simulink model "Rcontrol_veryold"  (Simulink 7.5)
settings: Solver=ode3  StartTime=0.0  StopTime=inf  FixedStep=SampleTime  RelTol=1e-3
undefined symbols (not defined in the file or in its folder): none, Rec, SampleTime, SDTV, videoinput
libraries: simulink x4, vipsnks x3, vipconversions x2, vipstatistics x1, viptextngfix x1, imaqlib x1, simulink_need_slupdate x1
settings Model: Creator=Duarte  LastModifiedBy=PC1
settings CodeAppCC: CustomSymbolStrType=$N$R$M_T
settings GRTTargetCC: TargetFunctionLibrary=NOT IN USE

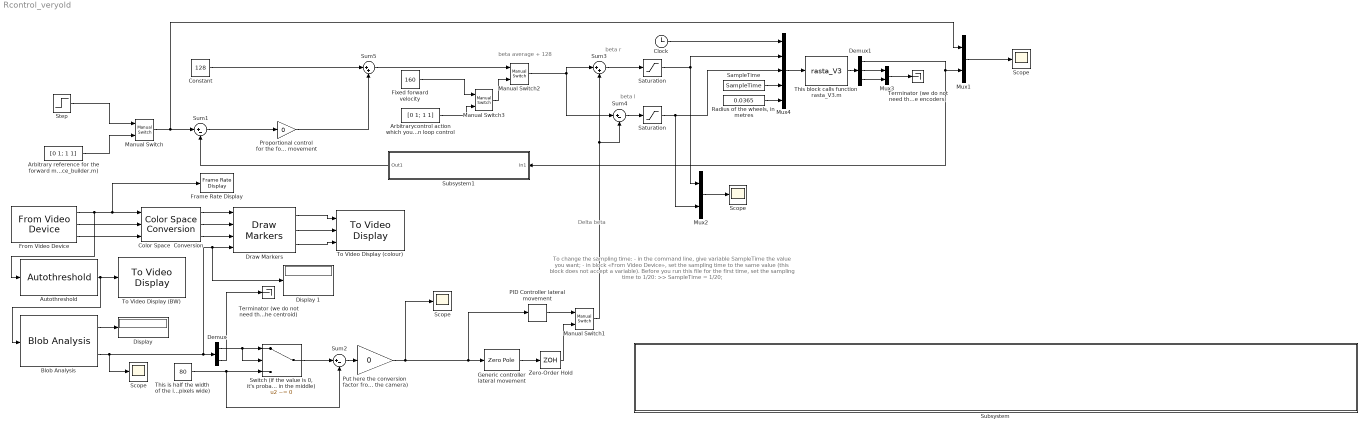
== system Rcontrol_veryold ==
  note: beta l
  note: beta r
  note: beta average + 128
  note: Delta beta
  note: To change the sampling time:
      | - in the command line, give variable SampleTime the value you want;
      | - in block «From Video Device», set the sampling time to the same value (this block does not accept a variable).
      | Before you run this file for the first time, set the sampling time to 1/20:
      |      >> SampleTime = 1/20;
  "Arbitrary reference for the forward movement, which you may change (use here the variable created by reference_builder.m)" : FromWorkspace  VariableName=[0 1; 1 1]  SampleTime=SampleTime
  Arbitrarycontrol action which you may use for open loop control : FromWorkspace  VariableName=[0 1; 1 1]  SampleTime=SampleTime
  Autothreshold : vipconversions/Autothreshold  DialogController=vipDDGCreate  DialogControllerArgs=DataTag0  operator=<=  threshOut=off  effMetricOut=off  userDefinedRange=off  umin=0  umax=255  outOfRngOpt=Warn and saturate  scaleThreshold=off  scaleFactor=1  P1Mode=Specify word length  P1WordLength=32  P1FracLength=30  P2Mode=Specify word length  P2WordLength=32  P2FracLength=22  P3Mode=Specify word length  P3WordLength=32  P3FracLength=14  P4Mode=Binary point scaling  P4WordLength=32  P4FracLength=15  Q1Mode=Specify word length  Q1WordLength=32  Q1FracLength=16  EMMode=Specify word length  EMWordLength=16  EMFracLength=14  roundingMode=Floor  overflowMode=off
  Blob Analysis : vipstatistics/Blob Analysis  Tag=vipblks_row_conv  DialogController=vipDDGCreate  DialogControllerArgs=DataTag1  area=on  centroid=on  bBox=off  majorAxis=off  minorAxis=off  angle=off  eccentricity=off  equivDiameterSq=off  extent=off  perimeter=off  maxBlobs=1  warnIfNumBlobsExceeded=off  isCount=off  useMinArea=off  minArea=0  useMaxArea=off  maxArea=intmax('uint32')  excludeBorderBlob=off  outDT=double  isOutVarDim=off  isFill=on  fillValues=-1  conn=8  isLabel=off  outputMode=Binary point scaling  outputWordLength=32  outputFracLength=16  firstCoeffMode=Binary point scaling  firstCoeffWordLength=16  firstCoeffFracLength=14  secondCoeffMode=Binary point scaling  secondCoeffWordLength=32  secondCoeffFracLength=16  accumMode=Binary point scaling  accumWordLength=32  accumFracLength=0  prodOutputMode=Binary point scaling  prodOutputWordLength=32  prodOutputFracLength=16  roundingMode=Floor  overflowMode=off
  Clock : Clock
      settings: Decimation=10
  Color Space  Conversion : vipconversions/Color Space  Conversion  conversion=Obsolete  conversionActive=Y'CbCr to R'G'B'  wp_str=D65  rec=Rec. 601 (SDTV)  sys=1125/60/2:1  imagePorts=Separate color signals
  Constant : Constant  Value=128
  Demux : Demux  Outputs=2
  Demux1 : Demux  Outputs=3
  "Display " : Display
  Display 1 : Display
  Draw Markers : viptextngfix/Draw Markers  DialogController=vipDDGCreate  DialogControllerArgs=DataTag2  shape=Circle  size=5  fill=off  fillClrSource=Specify via dialog  display=User-specified value  intensity=200  color=[200 0 0]  opacity=0.6  viewport=Entire image  antialiasing=off  inType=Obsolete  imagePorts=Separate color signals  prodOutputMode=Binary point scaling  prodOutputWordLength=32  prodOutputFracLength=14  memoryMode=Specify word length  memoryWordLength=16  memoryFracLength=15  roundingMode=Floor  overflowMode=off
  Fixed forward velocity : Constant  Value=160
  Frame Rate Display : vipsnks/Frame Rate Display  DialogController=vipDDGCreate  DialogControllerArgs=DataTag3  UpdateRate=10
  From Video Device : imaqlib/From Video Device  DialogController=imaqcreatedialog  DialogControllerArgs=DataTag5  DeviceMenu=winvideo 2 (USB2.0 PC CAMERA)  Device=winvideo 2 (USB2.0 PC CAMERA)  ObjConstructor=videoinput('winvideo', 2)  VideoFormatMenu=YUY2_160x120  VideoFormat=YUY2_160x120  VideoSource=input1  ROIPosition=[0 0 120 160]  EnableHWTrigger=off  TriggerConfiguration=none/none  SampleTime=1/8  OutputPortsMode=Separate color signals  DataType=single  CanDoHWTrigger=no  ReturnedColorSpace=YCbCr  BlockHandle=17.001  ROIWidth=160  ROIHeight=120
  Generic controller lateral movement : ZeroPole  Zeros=[-1]  Poles=[-2]  Gain=1/3
  Manual Switch : simulink/Signal Routing/Manual Switch  SystemSampleTime=-1  sw=0  action=0  varsize=off
  Manual Switch1 : simulink/Signal Routing/Manual Switch  SystemSampleTime=-1  sw=1  action=0  varsize=off
  Manual Switch2 : simulink/Signal Routing/Manual Switch  SystemSampleTime=-1  sw=1  action=0  varsize=off
  Manual Switch3 : simulink/Signal Routing/Manual Switch  SystemSampleTime=-1  sw=1  action=0  varsize=off
  Mux1 : Mux  Inputs=2
  Mux2 : Mux  Inputs=2
  Mux3 : Mux  Inputs=2
  Mux4 : Mux  Inputs=5
  PID Controller lateral movement : simulink_need_slupdate/PID Controller  SystemSampleTime=-1  P=0  I=0  D=0
  Proportional control for the forward movement : Gain  Gain=0
  Put here the conversion factor from pixels to rad (this is the gain of the camera) : Gain  Gain=0
  "Radius of the wheels, in metres" : Constant  Value=0.0365
  SampleTime : Constant  Value=SampleTime
  Saturation : Saturate  UpperLimit=255  LowerLimit=0
  "Saturation " : Saturate  UpperLimit=255  LowerLimit=0
  Scope : Scope
      settings: YMin=0.985  YMax=1  SaveName=DataFwd
  "Scope  " : Scope
      settings: YMin=0  YMax=85  SaveName=DataCentr
  "Scope   " : Scope
      settings: SaveName=DataCtrl
  "Scope     " : Scope
      settings: SaveName=DataRotation
  Step : Step  Time=0  SampleTime=SampleTime
  Subsystem : Subsystem
      settings: OpenFcn=|
      | % find what ports have been open
      | whatsopen = instrfind;
      | for k = 1 : length(whatsopen)
      |     if strcmp( whatsopen(k).Status , 'open' )
      |         % if there's an open port...
      |         fclose(whatsopen(k));
      |         % ...close it
      |     end
      | end
      | % now we know everything's closed
      mask Display: disp('Double-click this block to close all the open ports')
  Subsystem1 : Subsystem
  Sum1 : Sum  Inputs=|+-
  Sum2 : Sum  Inputs=|+-
  Sum3 : Sum  Inputs=|++
  Sum4 : Sum  Inputs=|+-
  Sum5 : Sum  Inputs=|++
  "Switch (if the value is 0, it's probably a mistake, so assume it's in the middle)" : Switch  Criteria=u2 ~= 0
  Terminator (we do not need the values from the encoders) : Terminator
  Terminator (we do not need the y coordinate of the centroid) : Terminator
  This block calls function rasta_V3.m : MATLABFcn  MATLABFcn=rasta_V3  Output1D=off  SampleTime=SampleTime
  This is half the width of the image (change this if your image is not 160 pixels wide) : Constant  Value=80
  To Video Display (BW) : vipsnks/To Video Display  DialogControllerArgs=DataTag6  inputType=Obsolete  imagePorts=One multidimensional signal  OutputDevice=On-screen video monitor  fullScreen=off  videoWindowX=44  videoWindowY=27  saveWindowSize=off  videoWindowWidth=160  videoWindowHeight=120  dataOrg=Column-major  openAtMdlStart=on  isWindowOpen=on
  To Video Display (colour) : vipsnks/To Video Display  DialogControllerArgs=DataTag7  inputType=Obsolete  imagePorts=Separate color signals  OutputDevice=On-screen video monitor  fullScreen=off  videoWindowX=220  videoWindowY=27  saveWindowSize=off  videoWindowWidth=160  videoWindowHeight=120  dataOrg=Column-major  openAtMdlStart=on  isWindowOpen=on
  "Zero-Order Hold " : ZeroOrderHold  SampleTime=SampleTime
  wires:
  Mux4/1 -> This block calls function rasta_V3.m/1
  Clock/1 -> Mux4/1
  Constant/1 -> Sum5/1
  Manual Switch/1 -> Mux1/1, Sum1/1
  Sum1/1 -> Proportional control for the forward movement/1
  Mux1/1 -> Scope/1
  Proportional control for the forward movement/1 -> Sum5/2
  From Video Device/1 -> Color Space  Conversion/1, Frame Rate Display/1, Autothreshold/1
  From Video Device/2 -> Color Space  Conversion/2
  From Video Device/3 -> Color Space  Conversion/3
  Blob Analysis/2 -> "Scope  "/1, Demux/1, Draw Markers/4, Display 1/1
  Blob Analysis/1 -> "Display "/1
  Color Space  Conversion/1 -> Draw Markers/1
  Color Space  Conversion/2 -> Draw Markers/2
  Color Space  Conversion/3 -> Draw Markers/3
  Draw Markers/2 -> To Video Display (colour)/2
  Draw Markers/3 -> To Video Display (colour)/3
  Demux/1 -> "Switch (if the value is 0, it's probably a mistake, so assume it's in the middle)"/2, "Switch (if the value is 0, it's probably a mistake, so assume it's in the middle)"/1
  Demux/2 -> Terminator (we do not need the y coordinate of the centroid)/1
  Draw Markers/1 -> To Video Display (colour)/1
  Manual Switch1/1 -> Sum4/2, Sum3/2
  This is half the width of the image (change this if your image is not 160 pixels wide)/1 -> Sum2/2, "Switch (if the value is 0, it's probably a mistake, so assume it's in the middle)"/3
  Sum4/1 -> "Saturation "/1
  Sum3/1 -> Saturation/1
  "Saturation "/1 -> Mux4/3, Mux2/2
  Saturation/1 -> Mux4/2, Mux2/1
  Sum2/1 -> Put here the conversion factor from pixels to rad (this is the gain of the camera)/1
  "Switch (if the value is 0, it's probably a mistake, so assume it's in the middle)"/1 -> Sum2/1
  PID Controller lateral movement/1 -> Manual Switch1/1
  Generic controller lateral movement/1 -> "Zero-Order Hold "/1
  "Zero-Order Hold "/1 -> Manual Switch1/2
  Manual Switch2/1 -> Sum3/1, Sum4/1
  Subsystem1/1(Out1) -> Sum1/2
  Sum5/1 -> Manual Switch2/1
  Fixed forward velocity/1 -> Manual Switch3/1
  Mux2/1 -> "Scope   "/1
  Autothreshold/1 -> To Video Display (BW)/1, Blob Analysis/1
  This block calls function rasta_V3.m/1 -> Demux1/1
  Demux1/2 -> Mux3/1
  Demux1/3 -> Mux3/2
  Mux3/1 -> Terminator (we do not need the values from the encoders)/1
  Demux1/1 -> Subsystem1/1(In1), Mux1/2
  Put here the conversion factor from pixels to rad (this is the gain of the camera)/1 -> "Scope     "/1, Generic controller lateral movement/1, PID Controller lateral movement/1
  Step/1 -> Manual Switch/1
  "Arbitrary reference for the forward movement, which you may change (use here the variable created by reference_builder.m)"/1 -> Manual Switch/2
  SampleTime/1 -> Mux4/4
  "Radius of the wheels, in metres"/1 -> Mux4/5
  Manual Switch3/1 -> Manual Switch2/2
  Arbitrarycontrol action which you may use for open loop control/1 -> Manual Switch3/2

== system Rcontrol_veryold/Subsystem ==

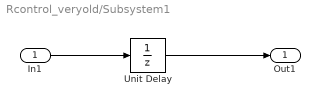
== system Rcontrol_veryold/Subsystem1 ==
  In1 : Inport
  Unit Delay : UnitDelay  SampleTime=SampleTime
  Out1 : Outport
  wires:
  In1/1 -> Unit Delay/1
  Unit Delay/1 -> Out1/1
